simulink model "curiosity_i2c_pitch_roll_yaw"  (R2025b)
settings: Solver=FixedStepDiscrete  StartTime=0.0  StopTime=inf  FixedStep=1e-3  RelTol=1e-3  EnableMultiTasking=on
undefined symbols (not defined in the file): A0, ADC, D10, D7, D8, D9, DiscIntNeverNeededParam, Max, MaxPer, ms, NumBits1, NumBits2, P1, P58, P59, Pin, Resol, s, Timer, us
libraries: MCHP_Blockset x18, simulink x17
(part 4 of 4)

== system curiosity_i2c_pitch_roll_yaw/MPU9250-AK8963 Accelerometers Gyrometers Magnetometers I2C Interface/Configure MPU-9250 ==
  Enable : EnablePort
  BUS I2C Configure AK8963 mag (MPU-9250) : MCHP_Blockset/BUS I2C/BUS I2C MASTER  I2CRef=2  I2C_IntPriority=5  I2Csequence_txt="Initial-Configuration$     ---     $Start$Write Address:{[0x0C]}    % AK8963 address$Write Data (x1)  Write:{[0x0A]}      % CNTL1$Write Data (x1)  Write:{[0x16]}      % 16bits-100Hz$Stop"  I2Csequence_num=[BFF0000000000000 40E0400000000000 41186A0000000000 41187A2B6F0EC141]$4070000000000000$[3FF0000000000000 40E0400000000000 410065D800000000 410065D9C7810E65]$[4040000000000000 0000000000000000 0000000000000000 4028000000000000]$[4050000000000000 3FF0000000000000 0000000000000000 4024000000000000]$[4050000000000000 3FF0000000000000 0000000000000000 4036000000000000]$[4000000000000000 40E0000000000000 40F86A0000000000 410065D9C7810E65]  InitialConfigurationNum=0  PIN_SDA_TXT=D8 / Pin[58]  PIN_SCL_TXT=D7 / Pin[57]  S_INPUT="[5  5]"  S_OUTPUT=[5]  S_INPUT_Size="[2  2]"  S_OUTPUT_Size=[4]  BlockingMode=off  SequenceCompleted=on  SampleTime=-1  MCHP_MASTERLINK=curiosity_i2c_pitch_roll_yaw/CuriosityPlatform Development Board dsPIC33AK128MC106 GP DIM/Microchip Master  MCHP_PORT={I2C 2 Clock}{SCL2}13:0:D7;{I2C 2 SDA}{SDA2}13:0:D8;  ORDERING=0
      settings: SourceProductName=MPLAB Device Blocks for Simulink
  BUS I2C Configure MPU-9250 : MCHP_Blockset/BUS I2C/BUS I2C MASTER  I2CRef=2  I2C_IntPriority=5  I2Csequence_txt="Initial-Configuration$     ---     $Start$Write Address:{MPU_9250.ADDR}    % MPU9250 I2C Address$Write Data (x1)  Write:{[0x6B]}      % ADR PWR_MGMT_1$Write Data (x1)  Write:{[0x01]}      % PWR_MGMT_1$Stop$Start$Write Address:{MPU_9250.ADDR}    % MPU9250 I2C Address$Write Data (x1)  Write:{[0x1A]}      % CONFIG reg addr$Write Data (x1)  Write:{MPU_9250.Config}      % CONFIG$Write Data (x1)  Write:{MPU_9250.Gyro_Config}      % GYRO_CONFIG$Write Data (x1)  Write:{MPU_9250.Accel_Config}      % ACCEL_CONFIG$Write Data (x1)  Write:{MPU_9250.Accel_Config2}      % ACCEL_CONFIG2$Stop"  I2Csequence_num=[BFF0000000000000 40E0400000000000 41186A0000000000 41187A2B6F0EC141]$4070000000000000$[3FF0000000000000 40E0200000000000 40F86A0000000000 40F866E066594CA2]$[4040000000000000 0000000000000000 0000000000000000 FFF8000000000000 4053400000000000 4054000000000000 4055400000000000 4057C00000000000 404C800000000000 4049000000000000 404A800000000000 4048000000000000 4047000000000000 4050400000000000 4051000000000000 4051000000000000 4054800000000000]$[4050000000000000 3FF0000000000000 0000000000000000 405AC00000000000]$[4050000000000000 3FF0000000000000 0000000000000000 3FF0000000000000]$[4000000000000000 40E0000000000000 41186A0000000000 4118666E3C87173F]$[3FF0000000000000 40E0200000000000 40F86A0000000000 40F866E066594CA2]$[4040000000000000 0000000000000000 0000000000000000 FFF8000000000000 4053400000000000 4054000000000000 4055400000000000 4057C00000000000 404C800000000000 4049000000000000 404A800000000000 4048000000000000 4047000000000000 4050400000000000 4051000000000000 4051000000000000 4054800000000000]$[4050000000000000 3FF0000000000000 0000000000000000 403A000000000000]$[4050000000000000 3FF0000000000000 0000000000000000 FFF8000000000000 4053400000000000 4054000000000000 4055400000000000 4057C00000000000 404C800000000000 4049000000000000 404A800000000000 4048000000000000 4047000000000000 4050C00000000000 405BC00000000000 405B800000000000 4059800000000000 405A400000000000 4059C00000000000]$[4050000000000000 3FF0000000000000 0000000000000000 FFF8000000000000 4053400000000000 4054000000000000 4055400000000000 4057C00000000000 404C800000000000 4049000000000000 404A800000000000 4048000000000000 4047000000000000 4051C00000000000 405E400000000000 405C800000000000 405BC00000000000 4057C00000000000 4050C00000000000 405BC00000000000 405B800000000000 4059800000000000 405A400000000000 4059C00000000000]$[4050000000000000 3FF0000000000000 0000000000000000 FFF8000000000000 4053400000000000 4054000000000000 4055400000000000 4057C00000000000 404C800000000000 4049000000000000 404A800000000000 4048000000000000 4047000000000000 4050400000000000 4058C00000000000 4058C00000000000 4059400000000000 405B000000000000 4057C00000000000 4050C00000000000 405BC00000000000 405B800000000000 4059800000000000 405A400000000000 4059C00000000000]$[4050000000000000 3FF0000000000000 0000000000000000 FFF8000000000000 4053400000000000 4054000000000000 4055400000000000 4057C00000000000 404C800000000000 4049000000000000 404A800000000000 4048000000000000 4047000000000000 4050400000000000 4058C00000000000 4058C00000000000 4059400000000000 405B000000000000 4057C00000000000 4050C00000000000 405BC00000000000 405B800000000000 4059800000000000 405A400000000000 4059C00000000000 4049000000000000]$[4000000000000000 40E0000000000000 40F86A0000000000 410065D9C7810E65]  InitialConfigurationNum=0  PIN_SDA_TXT=D8 / Pin[58]  PIN_SCL_TXT=D7 / Pin[57]  S_INPUT="[5  5]"  S_OUTPUT=[5]  S_INPUT_Size="[2  2]"  S_OUTPUT_Size=[4]  BlockingMode=off  SequenceCompleted=on  SampleTime=-1  MCHP_MASTERLINK=curiosity_i2c_pitch_roll_yaw/CuriosityPlatform Development Board dsPIC33AK128MC106 GP DIM/Microchip Master  MCHP_PORT={I2C 2 Clock}{SCL2}13:0:D7;{I2C 2 SDA}{SDA2}13:0:D8;  ORDERING=0
      settings: SourceProductName=MPLAB Device Blocks for Simulink
  Logical Operator : Logic  AllPortsSameDT=off  OutDataTypeStr=boolean
  Ok : Outport  InitialOutput=0  VectorParamsAs1DForOutWhenUnconnected=off
  wires:
  Logical Operator/1 -> Ok/1
  BUS I2C Configure MPU-9250/1 -> Logical Operator/1
  BUS I2C Configure AK8963 mag (MPU-9250)/1 -> Logical Operator/2

== system curiosity_i2c_pitch_roll_yaw/MPU9250-AK8963 Accelerometers Gyrometers Magnetometers I2C Interface/MPU-9250 ByPass I2C to AK8963 magnetometer Read IDs ==
  Enable : EnablePort
  MPU-9250 ByPass I2C to AK8963 magnetometer Read IDs : MCHP_Blockset/BUS I2C/BUS I2C MASTER  I2CRef=2  I2C_IntPriority=5  I2Csequence_txt="Initial-Configuration$     ---     $Start$Write Address:{MPU_9250.ADDR}    % MPU9250 I2C Address$Write Data (x1)  Write:{[0x75]}      % Who Am I (0x71)$Re-Start    % Re-Start when not followed with either Read or Write action rethrow Address$Write Address:{MPU_9250.ADDR}    % MPU9250 I2C Address$Read Data (x1)  Read:{ID MPU9250}    % ID= 0x71 (113)$Stop$Start$Write Address:{MPU_9250.ADDR}    % MPU9250 I2C Address$Write Data (x1)  Write:{[0x37]}      % INT_PIN_CFG$Write Data (x1)  Write:{[0x02]}      % I2C Pass_Through toward AK8963$Stop$Start$Write Address:{0x0C}    % AK8963 address$Write Data (x1)  Write:{[0x00]}      % ID$Re-Start$Write Address:{[0x0C]}    % AK8963 address$Read Data (x1)  Read:{ID AK8963}    % ID 0x48 (72)$Stop"  I2Csequence_num=[BFF0000000000000 40E0400000000000 41186A0000000000 41187A2B6F0EC141]$4070000000000000$[3FF0000000000000 40E0200000000000 40F86A0000000000 40F866E066594CA2]$[4040000000000000 0000000000000000 0000000000000000 FFF8000000000000 4053400000000000 4054000000000000 4055400000000000 4057C00000000000 404C800000000000 4049000000000000 404A800000000000 4048000000000000 4047000000000000 4050400000000000 4051000000000000 4051000000000000 4054800000000000]$[4050000000000000 3FF0000000000000 0000000000000000 405D400000000000]$[4008000000000000 40E0000000000000 40F86A0000000000 410065D9C7810E65]$[4040000000000000 0000000000000000 0000000000000000 FFF8000000000000 4053400000000000 4054000000000000 4055400000000000 4057C00000000000 404C800000000000 4049000000000000 404A800000000000 4048000000000000 4047000000000000 4050400000000000 4051000000000000 4051000000000000 4054800000000000]$[4060000000000000 3FF0000000000000]$[4000000000000000 40E0000000000000 40F86A0000000000 410065D9C7810E65]$[3FF0000000000000 40E0200000000000 40F86A0000000000 40F866E066594CA2]$[4040000000000000 0000000000000000 0000000000000000 FFF8000000000000 4053400000000000 4054000000000000 4055400000000000 4057C00000000000 404C800000000000 4049000000000000 404A800000000000 4048000000000000 4047000000000000 4050400000000000 4051000000000000 4051000000000000 4054800000000000]$[4050000000000000 3FF0000000000000 0000000000000000 404B800000000000]$[4050000000000000 3FF0000000000000 0000000000000000 4000000000000000]$[4000000000000000 40E0000000000000 40F86A0000000000 410065D9C7810E65]$[3FF0000000000000 40E0400000000000 410065D800000000 410065D9C7810E65]$[4040000000000000 0000000000000000 0000000000000000 4028000000000000]$[4050000000000000 3FF0000000000000 0000000000000000 0000000000000000]$[4008000000000000 40E0400000000000 410065D800000000 410065D9C7810E65]$[4040000000000000 0000000000000000 0000000000000000 4028000000000000]$[4060000000000000 3FF0000000000000]$[4000000000000000 40E0000000000000 40F86A0000000000 410065D9C7810E65]  InitialConfigurationNum=0  PIN_SDA_TXT=D8 / Pin[58]  PIN_SCL_TXT=D7 / Pin[57]  S_INPUT="[5  5]"  S_OUTPUT=[5]  S_INPUT_Size="[2  2]"  S_OUTPUT_Size=[4]  BlockingMode=off  SequenceCompleted=on  SampleTime=[0.1]  MCHP_MASTERLINK=curiosity_i2c_pitch_roll_yaw/CuriosityPlatform Development Board dsPIC33AK128MC106 GP DIM/Microchip Master  MCHP_PORT={I2C 2 Clock}{SCL2}13:0:D7;{I2C 2 SDA}{SDA2}13:0:D8;  ORDERING=0
      settings: SourceProductName=MPLAB Device Blocks for Simulink
  Ok : Outport  InitialOutput=0  VectorParamsAs1DForOutWhenUnconnected=off
  Id MPU9250 : Outport  Port=2  VectorParamsAs1DForOutWhenUnconnected=off
  "Id AK8963 " : Outport  Port=3  VectorParamsAs1DForOutWhenUnconnected=off
  wires:
  MPU-9250 ByPass I2C to AK8963 magnetometer Read IDs/1 -> Ok/1
  MPU-9250 ByPass I2C to AK8963 magnetometer Read IDs/2 -> Id MPU9250/1
  MPU-9250 ByPass I2C to AK8963 magnetometer Read IDs/3 -> "Id AK8963 "/1

== system curiosity_i2c_pitch_roll_yaw/MPU9250-AK8963 Accelerometers Gyrometers Magnetometers I2C Interface/Sample magnetometers on MPU-9250-AK8963 ==
  Enable : EnablePort
  BUS I2C Read Magnetometers @ 100Hz : MCHP_Blockset/BUS I2C/BUS I2C MASTER  I2CRef=2  I2C_IntPriority=5  I2Csequence_txt="Initial-Configuration$     ---     $Start$Write Address:{[0x0C]}    % AK8963 address$Write Data (x1)  Write:{[0x02]}      % Addr Start readding$Re-Start$Write Address:{[0x0C]}    % AK8963 address$Read Data (x1)  Read:{ST1}    % ST1$Read Data (x2)  Read:{MAG-X}    % MAG$Read Data (x2)  Read:{MAG-Y}    % MAG$Read Data (x2)  Read:{MAG-Z}    % MAG$Read Data (x1)  Read:{ST2}    % ST2 read required$Stop"  I2Csequence_num=[BFF0000000000000 40E0400000000000 41186A0000000000 41187A2B6F0EC141]$4070000000000000$[3FF0000000000000 40E0400000000000 410065D800000000 410065D9C7810E65]$[4040000000000000 0000000000000000 0000000000000000 4028000000000000]$[4050000000000000 3FF0000000000000 0000000000000000 4000000000000000]$[4008000000000000 40E0400000000000 410065D800000000 410065D9C7810E65]$[4040000000000000 0000000000000000 0000000000000000 4028000000000000]$[4060000000000000 3FF0000000000000]$[4060000000000000 4000000000000000]$[4060000000000000 4000000000000000]$[4060000000000000 4000000000000000]$[4060000000000000 3FF0000000000000]$[4000000000000000 40E0000000000000 40F86A0000000000 410065D9C7810E65]  InitialConfigurationNum=0  PIN_SDA_TXT=D8 / Pin[58]  PIN_SCL_TXT=D7 / Pin[57]  S_INPUT="[5  5]"  S_OUTPUT=[5]  S_INPUT_Size="[2  2]"  S_OUTPUT_Size=[4]  BlockingMode=off  SequenceCompleted=on  SampleTime=-1  MCHP_MASTERLINK=curiosity_i2c_pitch_roll_yaw/CuriosityPlatform Development Board dsPIC33AK128MC106 GP DIM/Microchip Master  MCHP_PORT={I2C 2 Clock}{SCL2}13:0:D7;{I2C 2 SDA}{SDA2}13:0:D8;  ORDERING=0
      settings: SourceProductName=MPLAB Device Blocks for Simulink
  Concat7 : Subsystem
  Concat8 : Subsystem
  Concat9 : Subsystem
  Ok : Outport  InitialOutput=0  VectorParamsAs1DForOutWhenUnconnected=off
  ST1 : Outport  Port=2  VectorParamsAs1DForOutWhenUnconnected=off
  MAG-X : Outport  Port=3  VectorParamsAs1DForOutWhenUnconnected=off
  MAX-Y : Outport  Port=4  VectorParamsAs1DForOutWhenUnconnected=off
  MAG-Z : Outport  Port=5  VectorParamsAs1DForOutWhenUnconnected=off
  ST2 : Outport  Port=6  VectorParamsAs1DForOutWhenUnconnected=off
  wires:
  BUS I2C Read Magnetometers @ 100Hz/6 -> ST2/1
  BUS I2C Read Magnetometers @ 100Hz/5 -> Concat9/1("[L H]")
  BUS I2C Read Magnetometers @ 100Hz/4 -> Concat8/1("[L H]")
  BUS I2C Read Magnetometers @ 100Hz/3 -> Concat7/1("[L H]")
  BUS I2C Read Magnetometers @ 100Hz/2 -> ST1/1
  BUS I2C Read Magnetometers @ 100Hz/1 -> Ok/1
  Concat7/1(HL) -> MAG-X/1  "U1 CH7"
  Concat9/1(HL) -> MAG-Z/1  "U1 CH9"
  Concat8/1(HL) -> MAX-Y/1  "U1 CH8"

== system curiosity_i2c_pitch_roll_yaw/MPU9250-AK8963 Accelerometers Gyrometers Magnetometers I2C Interface/Sample rate gyro and Accel on MPU-9250 ==
  Enable : EnablePort
  BUS I2C Gyro and Accel @ 1kHz : MCHP_Blockset/BUS I2C/BUS I2C MASTER  I2CRef=2  I2C_IntPriority=5  I2Csequence_txt="Initial-Configuration$     ---     $Update-Configuration$Start$Write Address:{MPU_9250.ADDR}    % MPU9250 I2C Address$Write Data (x1)  Write:{[0x3B]}      % ACCEL_XOUT_H$Re-Start    % Re-Start when not followed with either Read or Write action rethrow Address$Write Address:{MPU_9250.ADDR}    % MPU9250 I2C Address$Read Data (x2)  Read:{Ax}    % Accel Temp Gyro$Read Data (x2)  Read:{Ay}    % Accel Temp Gyro$Read Data (x2)  Read:{Ax}    % z$Read Data (x2)  Read:{Temp}    % Accel Temp Gyro$Read Data (x2)  Read:{Gx}    % Accel Temp Gyro$Read Data (x2)  Read:{Gy}    % Accel Temp Gyro$Read Data (x2)  Read:{Gz}    % Accel Temp Gyro$Stop$Update-Configuration"  I2Csequence_num=[BFF0000000000000 40E0400000000000 41186A0000000000 41187A2B6F0EC141]$4070000000000000$[0000000000000000 40E0400000000000 41186A0000000000 41186A0000000000]$[3FF0000000000000 40E0200000000000 40F86A0000000000 40F866E066594CA2]$[4040000000000000 0000000000000000 0000000000000000 FFF8000000000000 4053400000000000 4054000000000000 4055400000000000 4057C00000000000 404C800000000000 4049000000000000 404A800000000000 4048000000000000 4047000000000000 4050400000000000 4051000000000000 4051000000000000 4054800000000000]$[4050000000000000 3FF0000000000000 0000000000000000 404D800000000000]$[4008000000000000 40E0000000000000 40F86A0000000000 410065D9C7810E65]$[4040000000000000 0000000000000000 0000000000000000 FFF8000000000000 4053400000000000 4054000000000000 4055400000000000 4057C00000000000 404C800000000000 4049000000000000 404A800000000000 4048000000000000 4047000000000000 4050400000000000 4051000000000000 4051000000000000 4054800000000000]$[4060000000000000 4000000000000000]$[4060000000000000 4000000000000000]$[4060000000000000 4000000000000000]$[4060000000000000 4000000000000000]$[4060000000000000 4000000000000000]$[4060000000000000 4000000000000000]$[4060000000000000 4000000000000000]$[4000000000000000 40E0000000000000 40F86A0000000000 410065D9C7810E65]$[0000000000000000 40E0400000000000 41186A0000000000 4118666E3C87173F]  InitialConfigurationNum=0  PIN_SDA_TXT=D8 / Pin[58]  PIN_SCL_TXT=D7 / Pin[57]  S_INPUT="[5  5]"  S_OUTPUT=[5]  S_INPUT_Size="[2  2]"  S_OUTPUT_Size=[4]  BlockingMode=off  SequenceCompleted=on  SampleTime=-1  MCHP_MASTERLINK=curiosity_i2c_pitch_roll_yaw/CuriosityPlatform Development Board dsPIC33AK128MC106 GP DIM/Microchip Master  MCHP_PORT={I2C 2 Clock}{SCL2}13:0:D7;{I2C 2 SDA}{SDA2}13:0:D8;  ORDERING=0
      settings: SourceProductName=MPLAB Device Blocks for Simulink
  Concat : Subsystem
  Concat1 : Subsystem
  Concat2 : Subsystem
  Concat3 : Subsystem
  Concat4 : Subsystem
  Concat5 : Subsystem
  Concat6 : Subsystem
  Ok : Outport  InitialOutput=0  VectorParamsAs1DForOutWhenUnconnected=off
  Ax : Outport  Port=2  VectorParamsAs1DForOutWhenUnconnected=off
  Ay : Outport  Port=3  VectorParamsAs1DForOutWhenUnconnected=off
  Az : Outport  Port=4  VectorParamsAs1DForOutWhenUnconnected=off
  Temp : Outport  Port=5  VectorParamsAs1DForOutWhenUnconnected=off
  Gx : Outport  Port=6  VectorParamsAs1DForOutWhenUnconnected=off
  Gy : Outport  Port=7  VectorParamsAs1DForOutWhenUnconnected=off
  Gz : Outport  Port=8  VectorParamsAs1DForOutWhenUnconnected=off
  wires:
  BUS I2C Gyro and Accel @ 1kHz/8 -> Concat6/1("[H L]")
  BUS I2C Gyro and Accel @ 1kHz/7 -> Concat5/1("[H L]")
  BUS I2C Gyro and Accel @ 1kHz/6 -> Concat4/1("[H L]")
  BUS I2C Gyro and Accel @ 1kHz/5 -> Concat3/1("[H L]")
  BUS I2C Gyro and Accel @ 1kHz/4 -> Concat2/1("[H L]")
  BUS I2C Gyro and Accel @ 1kHz/3 -> Concat1/1("[H L]")
  BUS I2C Gyro and Accel @ 1kHz/2 -> Concat/1("[H L]")
  BUS I2C Gyro and Accel @ 1kHz/1 -> Ok/1
  Concat/1(HL) -> Ax/1  "U1 CH1"
  Concat3/1(HL) -> Temp/1
  Concat5/1(HL) -> Gy/1  "U1 CH5"
  Concat2/1(HL) -> Az/1  "U1 CH3"
  Concat4/1(HL) -> Gx/1  "U1 CH4"
  Concat6/1(HL) -> Gz/1  "U1 CH6"
  Concat1/1(HL) -> Ay/1  "U1 CH2"

== system curiosity_i2c_pitch_roll_yaw/MPU9250-AK8963 Accelerometers Gyrometers Magnetometers I2C Interface/Subsystem ==
  In1 : Inport
  In2 : Inport  Port=2
  In3 : Inport  Port=3
  In4 : Inport  Port=4
  In5 : Inport  Port=5
  In6 : Inport  Port=6
  In7 : Inport  Port=7
  Enable : EnablePort
  Out1 : Outport  VectorParamsAs1DForOutWhenUnconnected=off
  Out2 : Outport  Port=2  VectorParamsAs1DForOutWhenUnconnected=off
  Out3 : Outport  Port=3  VectorParamsAs1DForOutWhenUnconnected=off
  Out4 : Outport  Port=4  VectorParamsAs1DForOutWhenUnconnected=off
  Out5 : Outport  Port=5  VectorParamsAs1DForOutWhenUnconnected=off
  Out6 : Outport  Port=6  VectorParamsAs1DForOutWhenUnconnected=off
  Out7 : Outport  Port=7  VectorParamsAs1DForOutWhenUnconnected=off
  wires:
  In7/1 -> Out7/1
  In6/1 -> Out6/1
  In5/1 -> Out5/1
  In4/1 -> Out4/1
  In3/1 -> Out3/1
  In2/1 -> Out2/1
  In1/1 -> Out1/1

== system curiosity_i2c_pitch_roll_yaw/MPU9250-AK8963 Accelerometers Gyrometers Magnetometers I2C Interface/Subsystem1 ==
  In1 : Inport
  In2 : Inport  Port=2
  In3 : Inport  Port=3
  In4 : Inport  Port=4
  In5 : Inport  Port=5
  Enable : EnablePort
  Out1 : Outport  VectorParamsAs1DForOutWhenUnconnected=off
  Out2 : Outport  Port=2  VectorParamsAs1DForOutWhenUnconnected=off
  Out3 : Outport  Port=3  VectorParamsAs1DForOutWhenUnconnected=off
  Out4 : Outport  Port=4  VectorParamsAs1DForOutWhenUnconnected=off
  Out5 : Outport  Port=5  VectorParamsAs1DForOutWhenUnconnected=off
  wires:
  In1/1 -> Out1/1
  In2/1 -> Out2/1
  In3/1 -> Out3/1
  In4/1 -> Out4/1
  In5/1 -> Out5/1

== system curiosity_i2c_pitch_roll_yaw/MPU9250-AK8963 Accelerometers Gyrometers Magnetometers I2C Interface/open to configure MPU-9250 ==

== system curiosity_i2c_pitch_roll_yaw/CuriosityPlatform Development Board dsPIC33AK128MC106 GP DIM/Timing Analysis/Downsample Averaged2 ==
  note: DownSample & Average by changing data scaling
  In1 : Inport
  Compare To Constant : simulink/Logic and Bit Operations/Compare To Constant  relop===  const=1  OutDataTypeStr=boolean
  Counter Limited : simulink/Sources/Counter Limited  uplimit=DownSample-1  tsamp=-1
  Data Type Duplicate : DataTypeDuplicate
  Data Type Propagation : simulink/Signal Attributes/Data Type Propagation  PropDataType=fixdt(1, 16)  IfRefDouble=double  IfRefSingle=single  IsSigned=IsSigned1 or IsSigned2  NumBitsBase=NumBits1+NumBits2  NumBitsMult=1  NumBitsAdd=0  NumBitsAllowFinal=-1  PropScaling=2^-10  ValuesUsedBestPrec=[5 -7]  SlopeBase=Slope1  SlopeMult=1  SlopeAdd=0  BiasBase=Bias1  BiasMult=1  BiasAdd=0
  Data Type Propagation1 : simulink/Signal Attributes/Data Type Propagation  PropDataType=fixdt(1, 16)  IfRefDouble=double  IfRefSingle=single  IsSigned=IsSigned1 or IsSigned2  NumBitsBase=NumBits1+NumBits2  NumBitsMult=1  NumBitsAdd=0  NumBitsAllowFinal=-1  PropScaling=2^-10  ValuesUsedBestPrec=[5 -7]  SlopeBase=PosRange1  SlopeMult=1  SlopeAdd=0  BiasBase=Bias1  BiasMult=1  BiasAdd=0
  Discrete-Time Integrator : DiscreteIntegrator  IntegratorMethod=Accumulation: Backward Euler  gainval=1  ExternalReset=sampled level  SampleTime=-1  OutDataTypeStr=Inherit: Inherit via back propagation  ICPrevOutput=DiscIntNeverNeededParam  ICPrevScaledInput=DiscIntNeverNeededParam
  Gain : Gain  Gain=1/DownSample  OutDataTypeStr=Inherit: Inherit via back propagation
  Gain1 : Gain  Gain=1/DownSample  OutDataTypeStr=Inherit: Inherit via back propagation
  Rate Transition1 : RateTransition  Deterministic=off  OutPortSampleTime=[InputSampleTime * DownSample]
  Rate Transition3 : RateTransition  OutPortSampleTime=[InputSampleTime * DownSample]
  Terminator : Terminator
  Out1 : Outport  VectorParamsAs1DForOutWhenUnconnected=off
  wires:
  Gain1/1 -> Terminator/1, Data Type Propagation1/3
  Rate Transition1/1 -> Data Type Duplicate/1, Data Type Propagation1/1, Data Type Propagation1/2
  Gain/1 -> Out1/1, Data Type Duplicate/2
  Counter Limited/1 -> Compare To Constant/1
  Discrete-Time Integrator/1 -> Rate Transition3/1, Data Type Propagation/3
  Compare To Constant/1 -> Discrete-Time Integrator/2
  In1/1 -> Data Type Propagation/1, Data Type Propagation/2, Rate Transition1/1, Discrete-Time Integrator/1
  Rate Transition3/1 -> Gain/1, Gain1/1

== system curiosity_i2c_pitch_roll_yaw/MPU9250-AK8963 Accelerometers Gyrometers Magnetometers I2C Interface/Sample magnetometers on MPU-9250-AK8963/Concat7 ==
  "[L H]" : Inport
  Demux : Demux  Outputs=2
  Gain : Gain  Gain=2^8  OutDataTypeStr=int16
  Sum : Sum  RndMeth=Simplest  OutDataTypeStr=Inherit: Same as first input
  HL : Outport  VectorParamsAs1DForOutWhenUnconnected=off
  wires:
  Demux/2 -> Gain/1
  Demux/1 -> Sum/2
  Gain/1 -> Sum/1
  Sum/1 -> HL/1
  "[L H]"/1 -> Demux/1

== system curiosity_i2c_pitch_roll_yaw/MPU9250-AK8963 Accelerometers Gyrometers Magnetometers I2C Interface/Sample magnetometers on MPU-9250-AK8963/Concat8 ==
  "[L H]" : Inport
  Demux : Demux  Outputs=2
  Gain : Gain  Gain=2^8  OutDataTypeStr=int16
  Sum : Sum  RndMeth=Simplest  OutDataTypeStr=Inherit: Same as first input
  HL : Outport  VectorParamsAs1DForOutWhenUnconnected=off
  wires:
  "[L H]"/1 -> Demux/1
  Sum/1 -> HL/1
  Gain/1 -> Sum/1
  Demux/1 -> Sum/2
  Demux/2 -> Gain/1

== system curiosity_i2c_pitch_roll_yaw/MPU9250-AK8963 Accelerometers Gyrometers Magnetometers I2C Interface/Sample magnetometers on MPU-9250-AK8963/Concat9 ==
  "[L H]" : Inport
  Demux : Demux  Outputs=2
  Gain : Gain  Gain=2^8  OutDataTypeStr=int16
  Sum : Sum  RndMeth=Simplest  OutDataTypeStr=Inherit: Same as first input
  HL : Outport  VectorParamsAs1DForOutWhenUnconnected=off
  wires:
  Demux/2 -> Gain/1
  Demux/1 -> Sum/2
  Gain/1 -> Sum/1
  Sum/1 -> HL/1
  "[L H]"/1 -> Demux/1

== system curiosity_i2c_pitch_roll_yaw/MPU9250-AK8963 Accelerometers Gyrometers Magnetometers I2C Interface/Sample rate gyro and Accel on MPU-9250/Concat ==
  "[H L]" : Inport
  Demux : Demux  Outputs=2
  Gain : Gain  Gain=2^8  OutDataTypeStr=int16
  Sum : Sum  RndMeth=Simplest  OutDataTypeStr=Inherit: Same as first input
  HL : Outport  VectorParamsAs1DForOutWhenUnconnected=off
  wires:
  Demux/2 -> Sum/2
  Gain/1 -> Sum/1
  Demux/1 -> Gain/1
  Sum/1 -> HL/1
  "[H L]"/1 -> Demux/1

== system curiosity_i2c_pitch_roll_yaw/MPU9250-AK8963 Accelerometers Gyrometers Magnetometers I2C Interface/Sample rate gyro and Accel on MPU-9250/Concat1 ==
  "[H L]" : Inport
  Demux : Demux  Outputs=2
  Gain : Gain  Gain=2^8  OutDataTypeStr=int16
  Sum : Sum  RndMeth=Simplest  OutDataTypeStr=Inherit: Same as first input
  HL : Outport  VectorParamsAs1DForOutWhenUnconnected=off
  wires:
  "[H L]"/1 -> Demux/1
  Sum/1 -> HL/1
  Demux/1 -> Gain/1
  Gain/1 -> Sum/1
  Demux/2 -> Sum/2

== system curiosity_i2c_pitch_roll_yaw/MPU9250-AK8963 Accelerometers Gyrometers Magnetometers I2C Interface/Sample rate gyro and Accel on MPU-9250/Concat2 ==
  "[H L]" : Inport
  Demux : Demux  Outputs=2
  Gain : Gain  Gain=2^8  OutDataTypeStr=int16
  Sum : Sum  RndMeth=Simplest  OutDataTypeStr=Inherit: Same as first input
  HL : Outport  VectorParamsAs1DForOutWhenUnconnected=off
  wires:
  Demux/2 -> Sum/2
  Gain/1 -> Sum/1
  Demux/1 -> Gain/1
  Sum/1 -> HL/1
  "[H L]"/1 -> Demux/1

== system curiosity_i2c_pitch_roll_yaw/MPU9250-AK8963 Accelerometers Gyrometers Magnetometers I2C Interface/Sample rate gyro and Accel on MPU-9250/Concat3 ==
  "[H L]" : Inport
  Demux : Demux  Outputs=2
  Gain : Gain  Gain=2^8  OutDataTypeStr=int16
  Sum : Sum  RndMeth=Simplest  OutDataTypeStr=Inherit: Same as first input
  HL : Outport  VectorParamsAs1DForOutWhenUnconnected=off
  wires:
  "[H L]"/1 -> Demux/1
  Sum/1 -> HL/1
  Demux/1 -> Gain/1
  Gain/1 -> Sum/1
  Demux/2 -> Sum/2

== system curiosity_i2c_pitch_roll_yaw/MPU9250-AK8963 Accelerometers Gyrometers Magnetometers I2C Interface/Sample rate gyro and Accel on MPU-9250/Concat4 ==
  "[H L]" : Inport
  Demux : Demux  Outputs=2
  Gain : Gain  Gain=2^8  OutDataTypeStr=int16
  Sum : Sum  RndMeth=Simplest  OutDataTypeStr=Inherit: Same as first input
  HL : Outport  VectorParamsAs1DForOutWhenUnconnected=off
  wires:
  Demux/2 -> Sum/2
  Gain/1 -> Sum/1
  Demux/1 -> Gain/1
  Sum/1 -> HL/1
  "[H L]"/1 -> Demux/1

== system curiosity_i2c_pitch_roll_yaw/MPU9250-AK8963 Accelerometers Gyrometers Magnetometers I2C Interface/Sample rate gyro and Accel on MPU-9250/Concat5 ==
  "[H L]" : Inport
  Demux : Demux  Outputs=2
  Gain : Gain  Gain=2^8  OutDataTypeStr=int16
  Sum : Sum  RndMeth=Simplest  OutDataTypeStr=Inherit: Same as first input
  HL : Outport  VectorParamsAs1DForOutWhenUnconnected=off
  wires:
  "[H L]"/1 -> Demux/1
  Sum/1 -> HL/1
  Demux/1 -> Gain/1
  Gain/1 -> Sum/1
  Demux/2 -> Sum/2

== system curiosity_i2c_pitch_roll_yaw/MPU9250-AK8963 Accelerometers Gyrometers Magnetometers I2C Interface/Sample rate gyro and Accel on MPU-9250/Concat6 ==
  "[H L]" : Inport
  Demux : Demux  Outputs=2
  Gain : Gain  Gain=2^8  OutDataTypeStr=int16
  Sum : Sum  RndMeth=Simplest  OutDataTypeStr=Inherit: Same as first input
  HL : Outport  VectorParamsAs1DForOutWhenUnconnected=off
  wires:
  Demux/2 -> Sum/2
  Gain/1 -> Sum/1
  Demux/1 -> Gain/1
  Sum/1 -> HL/1
  "[H L]"/1 -> Demux/1

== matlab function curiosity_i2c_pitch_roll_yaw/Roll_&_Pitch_Yaw_Gyro/MATLAB Function ==
  data: y_now input; y_unwrap output
function y_unwrap = unwrap_block(y_now)

persistent y_prev initialized
if isempty(initialized)
    y_prev = y_now;     % initialize to first sample
    initialized = true;
end

d = y_now - y_prev;

H = 0.5;  % hysteresis in degrees
if d > 180 + H
    y_now = y_now - 360;
elseif d < -180 - H
    y_now = y_now + 360;
end

y_unwrap = y_now;
y_prev = y_unwrap;
end

== matlab function curiosity_i2c_pitch_roll_yaw/Subsystem/MATLAB Function ==
  data: y_now input; y_unwrap output
function y_unwrap = unwrap_block(y_now)

persistent y_prev initialized
if isempty(initialized)
    y_prev = y_now;     % initialize to first sample
    initialized = true;
end

d = y_now - y_prev;

H = 0.5;  % hysteresis in degrees
if d > 180 + H
    y_now = y_now - 360;
elseif d < -180 - H
    y_now = y_now + 360;
end

y_unwrap = y_now;
y_prev = y_unwrap;
end

== matlab function curiosity_i2c_pitch_roll_yaw/Yaw_Magnetometer/MATLAB Function ==
  data: y_now input; y_unwrap output
function y_unwrap = unwrap_block(y_now)

persistent y_prev initialized
if isempty(initialized)
    y_prev = y_now;     % initialize to first sample
    initialized = true;
end

d = y_now - y_prev;

H = 0.5;  % hysteresis in degrees
if d > 180 + H
    y_now = y_now - 360;
elseif d < -180 - H
    y_now = y_now + 360;
end

y_unwrap = y_now;
y_prev = y_unwrap;
end
